simulink model "gcu"  (R2025b)
settings: Solver=FixedStepAuto  StartTime=0.0  StopTime=10.0  RelTol=1e-3
undefined symbols (not defined in the file): controller, luen, quadcop, traj, Ts_gcs
settings Model: DataDictionary=project.sldd  Creator=Nick  LastModifiedBy=Nick

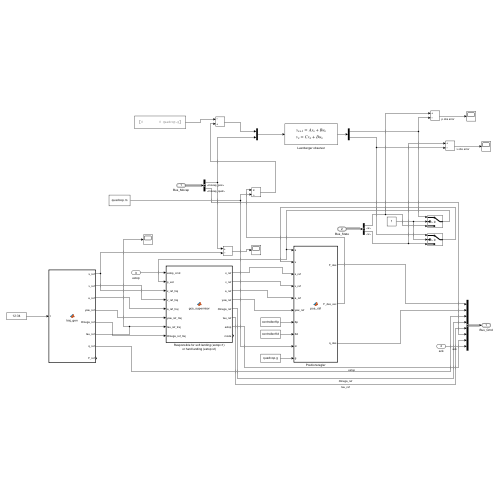
[thumbnail: Simulink's stored preview of the top-level diagram]
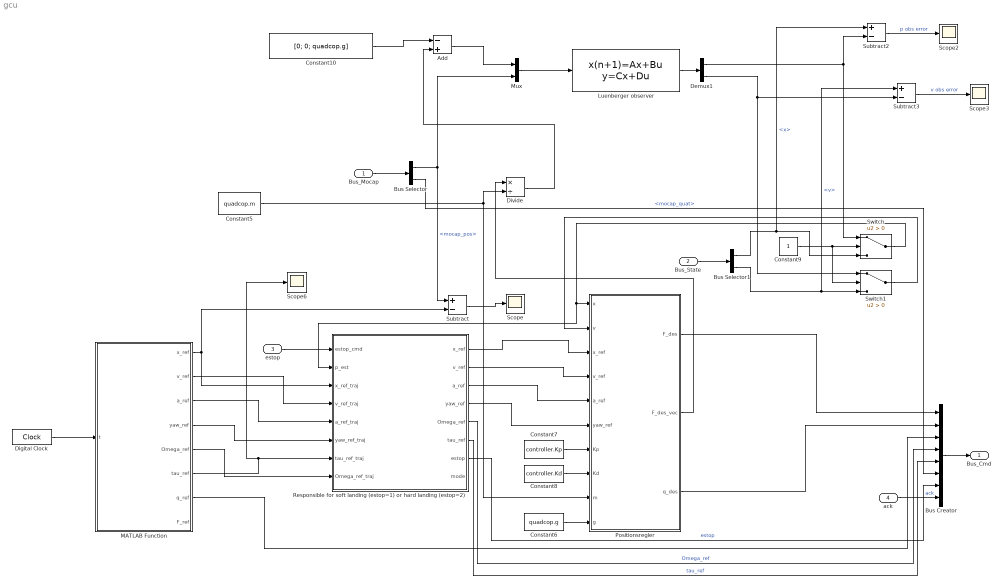
== system gcu ==
  Bus_Mocap : Inport  OutDataTypeStr=Bus: Bus_Mocap
  Bus_State : Inport  Port=2  OutDataTypeStr=Bus: Bus_State
  estop : Inport  Port=3  OutDataTypeStr=uint8
  ack : Inport  Port=4  OutDataTypeStr=boolean  PortDimensions=1
  Add : Sum  Inputs=-+
  Bus Creator : BusCreator  Inputs=8  OutDataTypeStr=Bus: Bus_Cmd
      settings: InheritFromInputs=off
  Bus Selector : BusSelector  OutputSignals=mocap_pos,mocap_quat
  Bus Selector1 : BusSelector  OutputSignals=x,v
  Constant10 : Constant  Value=[0; 0; quadcop.g]
  Constant5 : Constant  Value=quadcop.m
  Constant6 : Constant  Value=quadcop.g
  Constant7 : Constant  Value=controller.Kp
  Constant8 : Constant  Value=controller.Kd
  Constant9 : Constant
  Demux1 : Demux  Outputs=2
  Digital Clock : DigitalClock  SampleTime=Ts_gcs
  Divide : Product  Inputs=*/
  Luenberger observer : DiscreteStateSpace  A=luen.Ad  B=luen.Bd  C=luen.Cd  D=luen.Dd  InitialCondition=zeros(6,1)  SampleTime=Ts_gcs
  MATLAB Function : MATLAB Function  TreatAsAtomicUnit=on
  Mux : Mux  Inputs=2
  Positionsregler : MATLAB Function  TreatAsAtomicUnit=on
  Responsible for soft landing (estop=1) or hard landing (estop=2) : MATLAB Function  TreatAsAtomicUnit=on  SystemSampleTime=Ts_gcs
  Scope{,2..3,6} (4 alike) : Scope
      Scope settings: ActiveDisplayYMinimum=-0.059473818564182442  ActiveDisplayYMaximum=0.143243794641061
      Scope2 settings: ActiveDisplayYMinimum=-0.014392047751797402  ActiveDisplayYMaximum=0.012951900279030504  DataLoggingVariableName=ScopeData2
      Scope3 settings: ActiveDisplayYMinimum=-0.25096756656215152  ActiveDisplayYMaximum=0.3743542358396279  DataLoggingVariableName=ScopeData3
      Scope6 settings: ActiveDisplayYMinimum=-1  ActiveDisplayYMaximum=1  DataLoggingVariableName=ScopeData6
  Subtract : Sum  Inputs=+-
  Subtract2 : Sum  Inputs=+-
  Subtract3 : Sum  Inputs=+-
  Switch : Switch  Criteria=u2 > Threshold  SaturateOnIntegerOverflow=off  InputSameDT=off
  Switch1 : Switch  Criteria=u2 > Threshold  SaturateOnIntegerOverflow=off  InputSameDT=off
  Bus_Cmd : Outport  OutDataTypeStr=Bus: Bus_Cmd
  wires:
  Bus_Mocap/1 -> Bus Selector/1
  Bus Selector/1 -> Subtract/1, Mux/2  "<mocap_pos>"
  Constant5/1 -> Divide/2, Positionsregler/9(m)
  Bus_State/1 -> Bus Selector1/1
  Constant6/1 -> Positionsregler/10(g)
  Constant7/1 -> Positionsregler/7(Kp)
  Constant8/1 -> Positionsregler/8(Kd)
  Positionsregler/3(q_des) -> Bus Creator/2
  Bus Selector1/1 -> Subtract2/1, Switch/3  "<x>"
  Bus Selector1/2 -> Subtract3/1, Switch1/3  "<v>"
  Constant9/1 -> Switch1/2, Switch/2
  Switch/1 -> Responsible for soft landing (estop=1) or hard landing (estop=2)/2(p_est), Positionsregler/1(x)
  Switch1/1 -> Positionsregler/2(v)
  Demux1/1 -> Subtract2/2, Switch/1
  Subtract2/1 -> Scope2/1  "p obs error"
  Divide/1 -> Add/2
  Mux/1 -> Luenberger observer/1
  Luenberger observer/1 -> Demux1/1
  Demux1/2 -> Switch1/1, Subtract3/2
  Subtract3/1 -> Scope3/1  "v obs error"
  Constant10/1 -> Add/1
  Add/1 -> Mux/1
  MATLAB Function/1(x_ref) -> Responsible for soft landing (estop=1) or hard landing (estop=2)/3(x_ref_traj), Subtract/2
  MATLAB Function/2(v_ref) -> Responsible for soft landing (estop=1) or hard landing (estop=2)/4(v_ref_traj)
  MATLAB Function/3(a_ref) -> Responsible for soft landing (estop=1) or hard landing (estop=2)/5(a_ref_traj)
  MATLAB Function/4(yaw_ref) -> Responsible for soft landing (estop=1) or hard landing (estop=2)/6(yaw_ref_traj)
  Digital Clock/1 -> MATLAB Function/1(t)
  Bus Creator/1 -> Bus_Cmd/1
  MATLAB Function/7(q_ref) -> Bus Creator/3
  Bus Selector/2 -> Bus Creator/6  "<mocap_quat>"
  Positionsregler/1(F_des) -> Bus Creator/1
  Positionsregler/2(F_des_vec) -> Divide/1
  Subtract/1 -> Scope/1
  ack/1 -> Bus Creator/8  "ack"
  estop/1 -> Responsible for soft landing (estop=1) or hard landing (estop=2)/1(estop_cmd)
  Responsible for soft landing (estop=1) or hard landing (estop=2)/7(estop) -> Bus Creator/7  "estop"
  Responsible for soft landing (estop=1) or hard landing (estop=2)/1(x_ref) -> Positionsregler/3(x_ref)
  Responsible for soft landing (estop=1) or hard landing (estop=2)/2(v_ref) -> Positionsregler/4(v_ref)
  Responsible for soft landing (estop=1) or hard landing (estop=2)/3(a_ref) -> Positionsregler/5(a_ref)
  Responsible for soft landing (estop=1) or hard landing (estop=2)/4(yaw_ref) -> Positionsregler/6(yaw_ref)
  Responsible for soft landing (estop=1) or hard landing (estop=2)/6(tau_ref) -> Bus Creator/5  "tau_ref"
  Responsible for soft landing (estop=1) or hard landing (estop=2)/5(Omega_ref) -> Bus Creator/4  "Omega_ref"
  MATLAB Function/6(tau_ref) -> Responsible for soft landing (estop=1) or hard landing (estop=2)/7(tau_ref_traj), Scope6/1
  MATLAB Function/5(Omega_ref) -> Responsible for soft landing (estop=1) or hard landing (estop=2)/8(Omega_ref_traj)

== matlab function gcu/Positionsregler ==
  data: F_des output; x input; F_des_vec output; v input; x_ref input; v_ref input; a_ref input; yaw_ref input; Kp input; Kd input; m input; g input; q_des output
function [F_des, F_des_vec, q_des] = pos_ctrl(x, v, x_ref, v_ref, a_ref, yaw_ref, Kp, Kd, m, g)
%#codegen
% pos_ctrl PD-Positionsregler.
%   Erzeugt Sollschub F, Solllage q_ref und (fuer den Beobachter) die
%   kommandierte Inertialbeschleunigung a_cmd.
%
%   EIN-/AUSGAENGE:
%     x, v            : Position/Geschwindigkeit
%     x_d, v_d, a_d   : Solltrajektorie (Pos/Geschw/Beschl, inertial)
%     yaw_d           : Soll-Heading 
%     Kp, Kd          : 3x3-Gain-Matrizen
%     F               : Sollschubbetrag
%     q_ref           : Solllage-Quaternion
%     a_cmd           : kommandierte Inertialbeschleunigung (Beobachter-Eingang)

g_grav = [0; 0; g];

% --- Soll-Schubkraft (inertial): m*a_des + m*g_grav, a_des = a_d + Feedback ---
F_des_vec = m*(a_ref + g_grav - Kp*(x - x_ref) - Kd*(v - v_ref));

F_des = norm(F_des_vec);

% --- Kraft -> Lage: Koerper-z entlang F_des, Heading aus yaw_d ---
zb = F_des_vec / max(F_des, 1e-6); % gewuenschte Koerper-z in Inertial
xc = [cos(yaw_ref); sin(yaw_ref); 0];
yb = cross(zb, xc);  
yb = yb / max(norm(yb), 1e-6);
xb = cross(yb, zb);
Rd = [xb, yb, zb]; % R_{n<-b} (Koerper -> Inertial)
q_des = dcm2quat_local(Rd.');           

end

== matlab function gcu/MATLAB Function ==
  data: t input; x_ref output; v_ref output; a_ref output; yaw_ref output; Omega_ref output; tau_ref output; q_ref output; F_ref output; traj parameter; quadcop parameter
function [x_ref, v_ref, a_ref, yaw_ref, Omega_ref, tau_ref, q_ref, F_ref] = traj_gen(t, traj, quadcop)
%#codegen
% TRAJ_GEN  Minimum-Snap Punkt-zu-Punkt-Trajektorie
%
%   Liefert die Trajektorien für die flachen Ausgänge beim Arbeitspunktwechsel 
%   und daraus die Vorsteuerung. 
%
%   VERDRAHTUNG (2-DOF):
%     x_ref, v_ref, a_ref, yaw_ref  -> Positionsfolgeregler (äußere Kaskade)
%     q_ref, Omega_ref, tau_ff     -> Bus_Cmd   (reine Vorsteuerung)
%     F_ref   -> nur Debug/Verifikation (optional, unverbunden ok)
%
%   INPUTS
%     t    : Simulationszeit [s]  (z.B. Clock-Block)
%     traj : struct
%                  .P      3 x N      Wegpunkte 
%                  .yaw    1 x (N-1)  Yaw je Segment (konstant je Segment)
%                  .Tseg   1 x (N-1)  Bewegungsdauer je Segment 
%                  .Tdwell 1 x N      Rastdauer je Wegpunkt 
%            ANNAHME: N >= 2
%     quadcop  : struct 
%                  .m 
%                  .g  
%                  .J 
%
%   OUTPUTS
%     x_ref,v_ref,a_ref 3x1 Soll-Pos/Geschw/Beschl 
%     yaw_ref     1x1 Soll-Yaw 
%     Omega_ref   3x1 Vorsteuer-Drehrate (Body) 
%     tau_ff      3x1 Vorsteuer-Moment (Body) 
%     q_ref       4x1 nominelles Soll-Quaternion
%     F_ref       1x1 nomineller Schubbetrag = m*||a_d - g|| [N] -- Debug
%

    g_grav = [0; 0; quadcop.g];
    N = size(traj.P, 2);

    % ======================= Phase bestimmen =============================
    % Phasenfolge: dwell(1), move(1), dwell(2), move(2), ..., dwell(N)
    mode    = int8(2); % 0=Rast, 1=Bewegung, 2=End-Halt (Default)
    sel_wp  = N; % aktiver Wegpunkt (Rast/Halt)
    sel_seg = 1; % aktives Segment (Bewegung)
    tloc    = 0.0; % lokale Zeit in der Phase

    if t < 0
        mode = int8(0); 
        sel_wp = 1; 
        tloc = 0.0; % vor Start: WP1 halten
    else
        acc = 0.0;
        for i = 1:N
            Dd = traj.Tdwell(i); % Rast an WP i
            if (t >= acc) && (t < acc + Dd)
                mode = int8(0); 
                sel_wp = i; 
                tloc = t - acc; 
                break;
            end
            acc = acc + Dd;
            if i < N
                Tm = traj.Tseg(i); % Bewegung WP i -> i+1
                if (t >= acc) && (t < acc + Tm)
                    mode = int8(1); 
                    sel_seg = i; 
                    tloc = t - acc; 
                    break;
                end
                acc = acc + Tm;
            end
        end
        % kein break -> mode bleibt 2 (End-Halt an WP N)
    end

    % ===================== Trajektoriengenerierung =======================
    if mode == int8(1) % fliegt Trajektoriensegment ab
        k  = sel_seg;
        T  = traj.Tseg(k);
        tau = tloc / T;
        [s0,s1,s2,s3,s4] = restpoly(tau);
        D   = traj.P(:,k+1) - traj.P(:,k); % Differenz zwischen den Wegpunkten
        x_ref = traj.P(:,k) + D*s0;
        v_ref = D*s1 / T;
        a_ref = D*s2 / T^2;
        j_ref = D*s3 / T^3;
        s_ref = D*s4 / T^4;
        yaw_ref = traj.yaw(k);
    elseif mode == int8(0) % Rastpunkt
        x_ref = traj.P(:,sel_wp);
        v_ref = zeros(3,1);  
        a_ref = zeros(3,1);
        j_ref = zeros(3,1);
        s_ref = zeros(3,1);
        if sel_wp < N
            yaw_ref = traj.yaw(sel_wp);    % Yaw des kommenden Segments
        else
            yaw_ref = traj.yaw(N-1);
        end
    else % End-Halt
        x_ref = traj.P(:,N);
        v_ref = zeros(3,1);  
        a_ref = zeros(3,1);
        j_ref = zeros(3,1);
        s_ref = zeros(3,1);
        yaw_ref = traj.yaw(N-1);
    end

    % ================= Umrechnung von flachen Ausgängen und dessen Ableitungen 
    %               auf zugehörige Sollzustände =============================
    % Schubachse:  F*z_B = m*alpha,  alpha = a_ref - g_grav
    alpha = a_ref + g_grav;
    alphad = j_ref;
    alphadd = s_ref;

    n   = norm(alpha); % > 0 (nahe Hover ~ g)
    zB  = alpha / n;
    nd  = (alpha.'*alphad) / n;
    ndd = ((alphad.'*alphad) + (alpha.'*alphadd))/n - nd^2/n;
    zBd  = alphad/n - alpha*nd/n^2;
    zBdd = alphadd/n - 2*alphad*nd/n^2 - alpha*ndd/n^2 + 2*alpha*nd^2/n^3;

    % Heading (konstanter Yaw je Segment -> xC konstant, Ableitungen 0)
    xC = [cos(yaw_ref); sin(yaw_ref); 0];

    c   = cross(zB,   xC);
    cd  = cross(zBd,  xC);
    cdd = cross(zBdd, xC);
    nc   = norm(c); % Schutz: |zB x xC| ~ 1 nahe Hover
    if nc < 1e-6
        nc = 1e-6;
    end
    ncd  = (c.'*cd) / nc;
    ncdd = ((cd.'*cd) + (c.'*cdd))/nc - ncd^2/nc;
    yB   = c/nc;
    yBd  = cd/nc - c*ncd/nc^2;
    yBdd = cdd/nc - 2*cd*ncd/nc^2 - c*ncdd/nc^2 + 2*c*ncd^2/nc^3;

    xB   = cross(yB,   zB);
    xBd  = cross(yBd,  zB) + cross(yB,  zBd);
    xBdd = cross(yBdd, zB) + 2*cross(yBd, zBd) + cross(yB, zBdd);

    Rd   = [xB,   yB,   zB]; % = R_{n<-b}, Body -> Inertial
    Rdd  = [xBd,  yBd,  zBd]; % d/dt R_d
    Rddd = [xBdd, yBdd, zBdd]; % d2/dt2 R_d

    % [Omega]x = Rd' * Rdd <-> Rdd = Rd * [Omega]x
    Om_hat   = Rd.' * Rdd;
    Omega_ref = vee(0.5*(Om_hat - Om_hat.')); % force Om_hat back onto SO(3)
    % [Omegadot]x = Rd'*Rddd - [Omega]x^2
    Omd_hat  = Rd.' * Rddd - Om_hat*Om_hat;
    Omega_dot = vee(0.5*(Omd_hat - Omd_hat.'));

    tau_ref    = quadcop.J*Omega_dot + cross(Omega_ref, quadcop.J*Omega_ref);
    F_ref = quadcop.m * n;
    q_ref  = dcm2quat_local(Rd.');            % Rd' = R_{b<-n}
end

% =========================== Lokale Helfer ===============================

% function [s0,s1,s2,s3,s4] = restpoly(tau)
% % Minimum-Snap rest-to-rest Einheitsprofil 0->1 ueber tau in [0,1].
% % s und erste drei Ableitungen = 0 an beiden Enden (Snap != 0 an den Enden!).
%     if tau < 0  
%         tau = 0; 
%     elseif tau > 1 
%         tau = 1; 
%     end
%     t2=tau*tau; 
%     t3=t2*tau; 
%     t4=t3*tau; 
%     t5=t4*tau; 
%     t6=t5*tau; 
%     t7=t6*tau;
%     s0 =  35*t4 -  84*t5 +  70*t6 -  20*t7;
%     s1 = 140*t3 - 420*t4 + 420*t5 - 140*t6;     % ds/dtau
%     s2 = 420*t2 -1680*t3 +2100*t4 - 840*t5;     % d2s/dtau2
%     s3 = 840*tau-5040*t2 +8400*t3 -4200*t4;     % d3s/dtau3
%     s4 = 840    -10080*tau+25200*t2-16800*t3;   % d4s/dtau4
% end
function [s0,s1,s2,s3,s4] = restpoly(tau)
% Minimum-Crackle rest-to-rest Einheitsprofil 0->1 ueber tau in [0,1].
% s sowie die ersten VIER Ableitungen (v,a,j,s) = 0 an beiden Enden.
% -> Grad 9. Snap ist STETIG (==0) an den Enden => tau_ref springt
%    an Wegpunktuebergaengen nicht
    if tau < 0
        tau = 0;
    elseif tau > 1
        tau = 1;
    end
    t2 = tau*tau;
    t3 = t2*tau;
    t4 = t3*tau;
    t5 = t4*tau;
    t6 = t5*tau;
    t7 = t6*tau;
    t8 = t7*tau;
    t9 = t8*tau;
    s0 =   126*t5 -   420*t6 +   540*t7 -   315*t8 +  70*t9;
    s1 =   630*t4 -  2520*t5 +  3780*t6 -  2520*t7 + 630*t8;   % ds/dtau
    s2 =  2520*t3 - 12600*t4 + 22680*t5 - 17640*t6 + 5040*t7;  % d2s/dtau2
    s3 =  7560*t2 - 50400*t3 + 113400*t4 - 105840*t5 + 35280*t6; % d3s/dtau3
    s4 = 15120*tau - 151200*t2 + 453600*t3 - 529200*t4 + 211680*t5; % d4s/dtau4
end

function v = vee(S)
    v = [S(3,2); S(1,3); S(2,1)];
end

function q = dcm2quat_local(R)
% Shepperd, Skalar zuerst, R = Inertial->Koerper (R_{b<-n}).
% MUSS mit deiner Projektversion identisch sein (Vorzeichen!).
    r11=R(1,1); r22=R(2,2); r33=R(3,3);
    tr = r11+r22+r33;
    if tr > 0
        S = 2*sqrt(1+tr);
        q0 = 0.25*S;
        q1 = (R(2,3)-R(3,2))/S;
        q2 = (R(3,1)-R(1,3))/S;
        q3 = (R(1,2)-R(2,1))/S;
    elseif (r11 > r22) && (r11 > r33)
        S = 2*sqrt(1+r11-r22-r33);
        q0 = (R(2,3)-R(3,2))/S;
        q1 = 0.25*S;
        q2 = (R(1,2)+R(2,1))/S;
        q3 = (R(3,1)+R(1,3))/S;
    elseif r22 > r33
        S = 2*sqrt(1+r22-r11-r33);
        q0 = (R(3,1)-R(1,3))/S;
        q1 = (R(1,2)+R(2,1))/S;
        q2 = 0.25*S;
        q3 = (R(2,3)+R(3,2))/S;
    else
        S = 2*sqrt(1+r33-r11-r22);
        q0 = (R(1,2)-R(2,1))/S;
        q1 = (R(3,1)+R(1,3))/S;
        q2 = (R(2,3)+R(3,2))/S;
        q3 = 0.25*S;
    end
    q = [q0; q1; q2; q3];
    if q0 < 0, q = -q; end
    q = q / norm(q);
end

== matlab function gcu/Responsible for soft landing (estop=1) or hard landing (estop=2) ==
  data: estop_cmd input; x_ref output; p_est input; x_ref_traj input; v_ref_traj input; a_ref_traj input; yaw_ref_traj input; v_ref output; a_ref output; yaw_ref output; Omega_ref output; tau_ref output; estop output; mode output; tau_ref_traj input; supervisor parameter; Omega_ref_traj input
function [x_ref, v_ref, a_ref, yaw_ref, Omega_ref, tau_ref, estop, mode] = ...
        gcs_supervisor(estop_cmd, p_est, x_ref_traj, v_ref_traj, a_ref_traj, ...
                       yaw_ref_traj, tau_ref_traj, supervisor, Omega_ref_traj)
%#codegen
% GCS_SUPERVISOR Zustandsautomat
%
% Supervisor-MUX VOR pos_ctrl: waehlt die Sollwertquelle (Trajektorie vs.
% geregelter Soft-Land) und setzt das estop-Feld des Bus_Cmd aktiv. 
%
% ZUSTAENDE (mode):
%   0 NORMAL     : Sollwerte = Trajektorie estop=0
%   1 SOFT_LAND  : x/y eingefrieren, z-Ref rampt mit v_sink runter, v_ref=+v_sink,
%                  yaw halten. estop=1 (onboard sieht Soft-Land flag)
%   2 DISARMED   : Grund erreicht -> estop=2 -> onboard-Cutoff (rotors_cmd=0)
%   3 KILL       : Hard-Kill (estop_cmd==2 von ueberall) -> estop=2
%
%
% EINGAENGE:
%   estop_cmd       : uint8  Bediener-Wunsch  0 normal / 1 soft-land / 2 hard-kill
%   p_est           : 3x1    Positionsschaetzung [x;y;z] aus Luenberger
%   x_ref_traj      : 3x1    Trajektorien-Sollposition (Durchleitung in NORMAL)
%   v_ref_traj      : 3x1    Trajektorien-Sollgeschwindigkeit
%   a_ref_traj      : 3x1    Trajektorien-Sollbeschleunigung
%   yaw_ref_traj    : double Trajektorien-Soll-Yaw 
%   Omega_ref_traj  : 3x1    Trajektorien-Solldrehrate2
%   tau_ref_traj    : 3x1    Trajektorien-Sollmomente 
%   sup             : struct .v_sink .z_ground .disarm_margin .Ts
%
% AUSGAENGE (-> pos_ctrl bzw. Bus_Cmd):
%   x_ref, v_ref, a_ref : 3x1    selektierte Sollwerte fuer pos_ctrl
%   yaw_ref             : double selektierter Soll-Yaw
%   Omega_ref, tau_ref  : 3x1    Lage-Vorsteuerung 
%   estop               : uint8  0/1/2 -> Bus_Cmd.estop (Uplink)
%   mode                : uint8  Zustands-ID (Logging/Debug)

% --- Zustands-IDs ---
NORMAL = uint8(0);
SOFT_LAND = uint8(1);
DISARMED = uint8(2);
KILL = uint8(3);

persistent state x0 y0 yaw0 zref inited
if isempty(inited)
    state = NORMAL;
    x0 = 0.0;   
    y0 = 0.0;   
    yaw0 = 0.0;
    zref = 0.0;
    inited = true;
end

% --- Hard-Kill gewinnt immer, aus jedem Zustand ---
if estop_cmd == uint8(2)
    state = KILL;
end

% --- Transitionen + zustandslokale Aktualisierung ---
switch state
    case NORMAL
        if estop_cmd == uint8(1) % Soft-Land ausloesen
            state = SOFT_LAND;
            x0 = p_est(1); % Horizontalposition einfrieren
            y0 = p_est(2);
            yaw0 = yaw_ref_traj; % aktuellen Soll-Yaw halten
            zref = x_ref_traj(3); % z-Rampe startet auf aktueller Hoehe
        end

    case SOFT_LAND
        zref = zref - supervisor.v_sink * supervisor.Ts;
        if zref < supervisor.z_ground 
            zref = supervisor.z_ground;
        end
        % Disarm, sobald knapp ueber Grund (Mocap/Luenberger kennt Hoehe)
        if p_est(3) <= supervisor.z_ground + supervisor.disarm_margin
            state = DISARMED;
        end

    case DISARMED
        % terminal: estop=2 nullt onboard die Motoren

    otherwise % KILL
        % terminal
end

% --- Ausgangs-Mux nach Zustand ---
switch state
    case NORMAL
        x_ref   = x_ref_traj;
        v_ref   = v_ref_traj;
        a_ref   = a_ref_traj;
        yaw_ref = yaw_ref_traj;
        Omega_ref = Omega_ref_traj;   
        tau_ref   = tau_ref_traj;
        estop   = uint8(0);

    case SOFT_LAND
        x_ref   = [x0; y0; zref];       
        v_ref   = [0.0; 0.0; -supervisor.v_sink];
        a_ref   = [0.0; 0.0; 0.0];
        yaw_ref = yaw0;
        Omega_ref = [0.0; 0.0; 0.0];       
        tau_ref   = [0.0; 0.0; 0.0];
        estop   = uint8(1);

    case DISARMED % on-board-kill übernimmt
        x_ref   = [x0; y0; zref];
        v_ref   = [0.0; 0.0; supervisor.v_sink];
        a_ref   = [0.0; 0.0; 0.0];
        yaw_ref = yaw0;
        Omega_ref = [0.0; 0.0; 0.0];
        tau_ref   = [0.0; 0.0; 0.0];
        estop   = uint8(2);              

    otherwise % KILL
        x_ref   = [x0; y0; zref];                
        v_ref   = [0.0; 0.0; -supervisor.v_sink];
        a_ref   = [0.0; 0.0; 0.0];
        yaw_ref = yaw0;
        Omega_ref = [0.0; 0.0; 0.0];
        tau_ref   = [0.0; 0.0; 0.0];
        estop   = uint8(2);
end

mode = state;
end
